simulink model "rocket_flight_model"  (R2024b)
settings: Solver=ode4  StartTime=0.0  StopTime=10000  FixedStep=0.001  RelTol=1e-3
undefined symbols (not defined in the file): A, A_par, c, Cd, Fuel, G, h0, h_par, k, M, m, mFuel, Mol, p0, R, rGnd, s, Tair, v0, Vol
libraries: simulink_extras x1
settings Model: Creator=norbe  LastModifiedBy=norbe

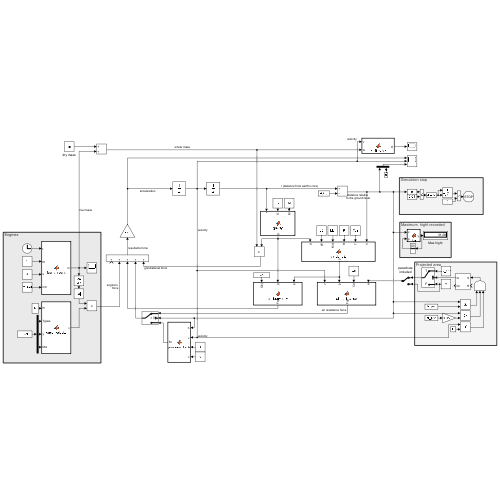
[thumbnail: Simulink's stored preview of the top-level diagram]
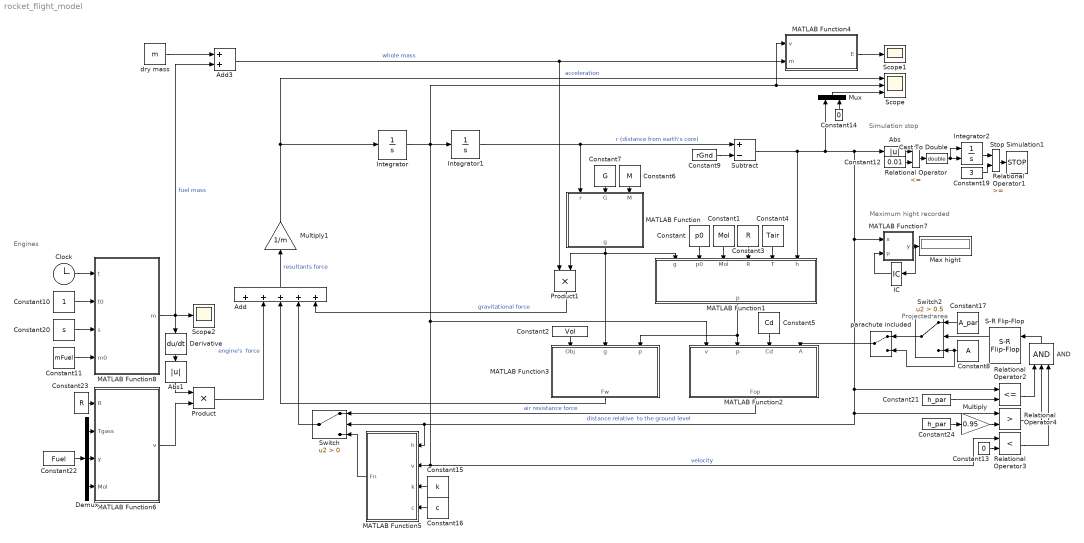
== system rocket_flight_model ==
  note: Maximum hight recorded
  note: Engines
  note: Projected area
  note: Simulation stop
  AND : Logic  Inputs=3  IconShape=distinctive  AllPortsSameDT=off  OutDataTypeStr=boolean
  Abs : Abs  SaturateOnIntegerOverflow=off
  Abs1 : Abs  SaturateOnIntegerOverflow=off
  Add : Sum  Inputs=+++++
  Add3 : Sum
  Cast To Double : DataTypeConversion  OutDataTypeStr=double  SaturateOnIntegerOverflow=off  RndMeth=Floor
  Clock : Clock
  Constant : Constant  Value=p0
  Constant1 : Constant  Value=Mol
  Constant10 : Constant
  Constant11 : Constant  Value=mFuel
  Constant12 : Constant  Value=0.01
  Constant13 : Constant  Value=0
  Constant14 : Constant  Value=0
  Constant15 : Constant  Value=k
  Constant16 : Constant  Value=c
  Constant17 : Constant  Value=A_par
  Constant19 : Constant  Value=3
  Constant2 : Constant  Value=Vol
  Constant20 : Constant  Value=s
  Constant21 : Constant  Value=h_par
  Constant22 : Constant  Value=Fuel
  Constant23 : Constant  Value=R
  Constant24 : Constant  Value=h_par
  Constant3 : Constant  Value=R
  Constant4 : Constant  Value=Tair
  Constant5 : Constant  Value=Cd
  Constant6 : Constant  Value=M
  Constant7 : Constant  Value=G
  Constant8 : Constant  Value=A
  Constant9 : Constant  Value=rGnd
  Demux : Demux  Outputs=3
  Derivative : Derivative
  IC : InitialCondition  Value=0
  Integrator : Integrator  InitialCondition=v0
  Integrator1 : Integrator  InitialCondition=rGnd+h0
  Integrator2 : Integrator  ExternalReset=falling
  MATLAB Function : MATLAB Function  TreatAsAtomicUnit=on
  MATLAB Function1 : MATLAB Function  TreatAsAtomicUnit=on
  MATLAB Function2 : MATLAB Function  TreatAsAtomicUnit=on
  MATLAB Function3 : MATLAB Function  TreatAsAtomicUnit=on
  MATLAB Function4 : MATLAB Function  TreatAsAtomicUnit=on
  MATLAB Function5 : MATLAB Function  TreatAsAtomicUnit=on
  MATLAB Function6 : MATLAB Function  TreatAsAtomicUnit=on
  MATLAB Function7 : MATLAB Function  TreatAsAtomicUnit=on
  MATLAB Function8 : MATLAB Function  TreatAsAtomicUnit=on
  Max hight : Display
  Multiply : Gain  Gain=0.95
  Multiply1 : Gain  Gain=1/m
  Mux : Mux  Inputs=2
  Product : Product
  Product1 : Product
  Relational Operator : RelationalOperator  Operator=<=  OutDataTypeStr=boolean  RndMeth=Simplest  InputSameDT=off
  Relational Operator1 : RelationalOperator  OutDataTypeStr=boolean  RndMeth=Simplest  InputSameDT=off
  Relational Operator2 : RelationalOperator  Operator=<=  OutDataTypeStr=boolean  RndMeth=Simplest  InputSameDT=off
  Relational Operator3 : RelationalOperator  Operator=<  OutDataTypeStr=boolean  RndMeth=Simplest  InputSameDT=off
  Relational Operator4 : RelationalOperator  Operator=>  OutDataTypeStr=boolean  RndMeth=Simplest  InputSameDT=off
  S-R Flip-Flop : simulink_extras/Flip Flops/S-R Flip-Flop  initial_condition=0
  Scope : Scope  NumInputPorts=3
  Scope1 : Scope
  Scope2 : Scope
  Stop Simulation1 : Stop
  Subtract : Sum  Inputs=+-
  Switch : Switch  Criteria=u2 > Threshold  SaturateOnIntegerOverflow=off  InputSameDT=off
  Switch2 : Switch  Criteria=u2 > Threshold  Threshold=0.5  SaturateOnIntegerOverflow=off  InputSameDT=off
  dry mass : Constant  Value=m
  parachute included : ManualSwitch
  wires:
  Integrator1/1 -> Subtract/1, MATLAB Function/1(r)  "r (distance from earth's core)"
  Constant1/1 -> MATLAB Function1/3(Mol)
  Constant/1 -> MATLAB Function1/2(p0)
  MATLAB Function/1(g) -> Product1/2, MATLAB Function1/1(g), MATLAB Function3/2(g)
  Constant3/1 -> MATLAB Function1/4(R)
  Constant4/1 -> MATLAB Function1/5(T)
  Constant7/1 -> MATLAB Function/2(G)
  Constant6/1 -> MATLAB Function/3(M)
  Constant5/1 -> MATLAB Function2/3(Cd)
  Constant9/1 -> Subtract/2
  Multiply1/1 -> Scope/1, Integrator/1  "acceleration"
  MATLAB Function1/1(p) -> MATLAB Function3/3(p), MATLAB Function2/2(p)
  MATLAB Function2/1(Fop) -> Switch/1  "air resistance force"
  Add/1 -> Multiply1/1  "resultants force"
  Switch/1 -> Add/4
  MATLAB Function5/1(Fn) -> Switch/3
  Subtract/1 -> Abs/1, MATLAB Function7/1(x), MATLAB Function5/1(h), Switch/2, Relational Operator4/1, Relational Operator2/1, Mux/1, MATLAB Function1/6(h)  "distance relative  to the ground level"
  Constant15/1 -> MATLAB Function5/3(k)
  Constant16/1 -> MATLAB Function5/4(c)
  MATLAB Function4/1(E) -> Scope1/1
  Integrator/1 -> MATLAB Function5/2(v), Relational Operator3/1, MATLAB Function2/1(v), MATLAB Function4/1(v), Scope/2, Integrator1/1  "velocity"
  Relational Operator/1 -> Cast To Double/1
  Cast To Double/1 -> Integrator2/2, Integrator2/1
  Relational Operator1/1 -> Stop Simulation1/1
  IC/1 -> MATLAB Function7/2(p)
  MATLAB Function7/1(y) -> Max hight/1, IC/1
  MATLAB Function6/1(v) -> Product/2
  Constant23/1 -> MATLAB Function6/1(R)
  Demux/3 -> MATLAB Function6/4(Mol)
  Demux/2 -> MATLAB Function6/3(y)
  Demux/1 -> MATLAB Function6/2(Tgass)
  Add3/1 -> MATLAB Function4/2(m), Product1/1  "whole mass"
  dry mass/1 -> Add3/1
  MATLAB Function8/1(m) -> Scope2/1, Derivative/1, Add3/2  "fuel mass"
  Clock/1 -> MATLAB Function8/1(t)
  Constant10/1 -> MATLAB Function8/2(t0)
  Constant11/1 -> MATLAB Function8/4(m0)
  Constant20/1 -> MATLAB Function8/3(s)
  Product/1 -> Add/2  "engine's  force"
  Derivative/1 -> Abs1/1
  Abs1/1 -> Product/1
  Product1/1 -> Add/5  "gravitational force"
  Mux/1 -> Scope/3
  Constant14/1 -> Mux/2
  Abs/1 -> Relational Operator/1
  Constant12/1 -> Relational Operator/2
  Integrator2/1 -> Relational Operator1/1
  Constant19/1 -> Relational Operator1/2
  Constant2/1 -> MATLAB Function3/1(Obj)
  MATLAB Function3/1(Fw) -> Add/3
  Constant22/1 -> Demux/1
  Constant8/1 -> parachute included/2, Switch2/3
  parachute included/1 -> MATLAB Function2/4(A)
  Multiply/1 -> Relational Operator4/2
  Constant24/1 -> Multiply/1
  Relational Operator4/1 -> AND/2
  Relational Operator2/1 -> AND/1
  Constant21/1 -> Relational Operator2/2
  Constant13/1 -> Relational Operator3/2
  Relational Operator3/1 -> AND/3
  AND/1 -> S-R Flip-Flop/1
  Switch2/1 -> parachute included/1
  S-R Flip-Flop/1 -> Switch2/2
  Constant17/1 -> Switch2/1

== matlab function rocket_flight_model/MATLAB Function1 ==
  data: g input; p0 input; Mol input; R input; T input; h input; p output
function p = air_density(g,p0,Mol,R,T,h)
p = p0*exp(-Mol*g*h/(R*T));

== matlab function rocket_flight_model/MATLAB Function ==
  data: r input; g output; G input; M input
function g = gravity(r,G,M)
g = -G*M/r^2;

== matlab function rocket_flight_model/MATLAB Function2 ==
  data: v input; Fop output; p input; Cd input; A input
function Fop = air_resistance(v,p,Cd,A)
Fop = 0.5*p*A*Cd*v^2;

== matlab function rocket_flight_model/MATLAB Function3 ==
  data: Obj input; g input; p input; Fw output
function Fw = air_buoyancy(Obj,g,p)
Fw = -p*g*Obj;

== matlab function rocket_flight_model/MATLAB Function4 ==
  data: v input; m input; E output
function E = KinEnergy(v,m)
E = 0.5*m*v^2;

== matlab function rocket_flight_model/MATLAB Function5 ==
  data: h input; v input; k input; Fn output; c input
function Fn = pressure_force(h,v,k,c)

Fn = -k*h-c*v;

== matlab function rocket_flight_model/MATLAB Function6 ==
  data: R input; v output; Tgass input; y input; Mol input
function v = gass_velocity(R,Tgass,y,Mol)
v = sqrt(2*y/(y-1)*R*Tgass/Mol);

== matlab function rocket_flight_model/MATLAB Function7 ==
  data: x input; y output; p input
function y = fcn(x,p)
if x>p
    y = x;
else
    y = p;
end

== matlab function rocket_flight_model/MATLAB Function8 ==
  data: t input; t0 input; s input; m output; m0 input
function m = fuel_amount(t,t0,s,m0)
if t <= t0
    m = m0;
else 
    mp = m0 -(t-t0)*s;
    if mp >= 0
        m = mp;
    else
    m = 0;
    end
end
